simulink model "lab3a"  (R2014b)
settings: Solver=ode45  StartTime=0.0  StopTime=10.0  RelTol=1e-3
libraries: powerlib x3
settings Model: Creator=angli  LastModifiedBy=angli

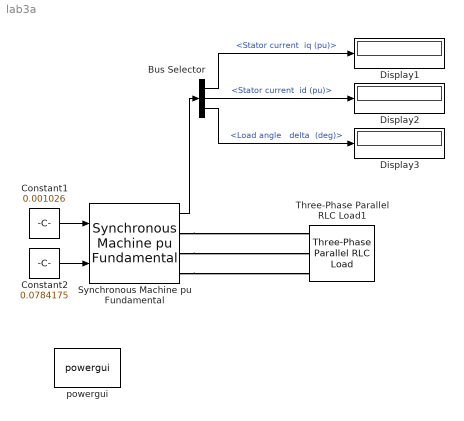
== system lab3a ==
  Bus Selector : BusSelector  OutputSignals="dq0 components.Stator current  iq (pu),dq0 components.Stator current  id (pu),Load angle   delta  (deg)"
  Constant1 : Constant  Value=0.001026
  Constant2 : Constant  Value=0.0784175
  Display1 : Display
  Display2 : Display
  Display3 : Display
  Synchronous Machine pu Fundamental : powerlib/Machines/Synchronous Machine pu Fundamental  PresetModel=No  MechanicalLoad=Mechanical power Pm  ShowDetailedParameters=on  RotorType=Salient-pole  Units=per unit fundamental parameters  MeasurementBus=off  NominalParameters="[100E6  11E3   50]"  Stator="[ 2.85E-03  0.15 1.3860  1.3440]"  Field="[ 0.0006  0.165]"  Dampers2=[0.0652, 0.5134, 0.0287, 0.2553, 7.765e-3, 0.9167 ]  Dampers1="[ 1.17E-02  0.182  1.97E-02  0.384 ]"  Mechanical=[ 3.7 0 20]  PolePairs=20  InitialConditions=[0 -89.0544 0.6 0.6 0.6 90 -30 -150 0.0784175]  SetSaturation=off  Saturation=[0.6404,0.7127,0.8441,0.9214,0.9956,1.082,1.19,1.316,1.457;0.7,0.7698,0.8872,0.9466,0.9969,1.046,1.1,1.151,1.201]  LoadFlowParameters=[2 0 0 0 0]  TsPowergui=0  TsBlock=-1  IterativeModel=Trapezoidal non iterative  BusType=PV  Pref=0  Qref=0  Qmin=-inf  Qmax=inf  PLF=0  QLF=0
  Three-Phase Parallel RLC Load1 : powerlib/Elements/Three-Phase Parallel RLC Load  LConnTagsString=A|B|C  Configuration=Y (grounded)  NominalVoltage=11E3  NominalFrequency=50  ActivePower=0  InductivePower=0  CapacitivePower=60e6  Measurements=None  LoadType=constant Z
  powergui : powerlib/powergui  Priority=1  SimulationMode=Phasor  SolverType=Tustin/Backward Euler (TBE)  SampleTime=50e-6  frequency=50  SPID=off  DisableSnubberDevices=off  DisableRonSwitches=off  DisableVfSwitches=off  SwTol=0  DisplayEquations=off  Interpol=off  methode=off  Ts=100  frequencyindice=50  Pbase=100e6  ErrMax=1e-4  Iterations=50  UnitsV=V  UnitsW=W  FunctionMessages=off  echomessages=off  HookPort=off  EnableUseOfTLC=off  x0status=blocks  RestoreLinks=warning  ResistiveCurrentMeasurement=off  Frange=[0:2:500]  Ylog=off  Xlog=on  ShowGrid=off  save=off  variable=ZData  structure=0  ZoomFFT=off  StartTime=0.0  cycles=1  DisplayStyle=1  fundamental=60  FreqAxis=off  MaxFrequency=1000  frequencyindicesteady=1  RmsSteady=1  display=off
  wires:
  Constant2/1 -> Synchronous Machine pu Fundamental/2
  Constant1/1 -> Synchronous Machine pu Fundamental/1
  Synchronous Machine pu Fundamental/1 -> Bus Selector/1
  Bus Selector/3 -> Display3/1  "<Load angle   delta  (deg)>"
  Bus Selector/2 -> Display2/1  "<Stator current  id (pu)>"
  Bus Selector/1 -> Display1/1  "<Stator current  iq (pu)>"
  connections:
  Synchronous Machine pu Fundamental/RConn1 -- Three-Phase Parallel RLC Load1/LConn1
  Synchronous Machine pu Fundamental/RConn2 -- Three-Phase Parallel RLC Load1/LConn2
  Synchronous Machine pu Fundamental/RConn3 -- Three-Phase Parallel RLC Load1/LConn3
